simulink model "Motor_model"  (R2024b)
settings: Solver=FixedStepDiscrete  StartTime=0.0  StopTime=10  FixedStep=0.001  RelTol=1e-3
settings Model: Creator=divg2  LastModifiedBy=divg2
settings RTWCC: GPUComputeCapability=3.5

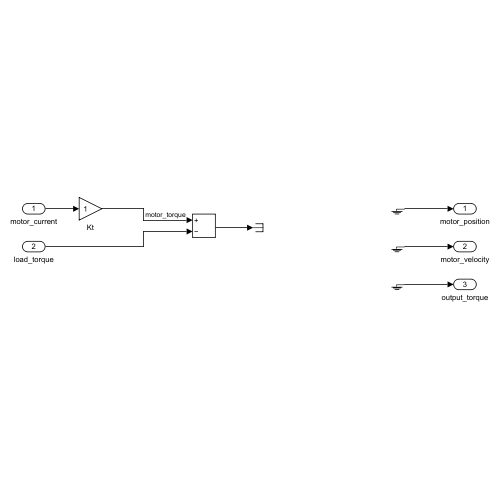
[thumbnail: Simulink's stored preview of the top-level diagram]
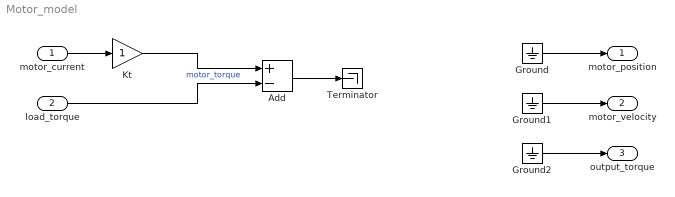
== system Motor_model ==
  motor_current : Inport
  load_torque : Inport  Port=2
  Add : Sum  Inputs=+-
  Ground : Ground
  Ground1 : Ground
  Ground2 : Ground
  Kt : Gain
  Terminator : Terminator
  motor_position : Outport
  motor_velocity : Outport  Port=2
  output_torque : Outport  Port=3
  wires:
  motor_current/1 -> Kt/1
  Ground/1 -> motor_position/1
  Ground1/1 -> motor_velocity/1
  Ground2/1 -> output_torque/1
  Kt/1 -> Add/1  "motor_torque"
  load_torque/1 -> Add/2
  Add/1 -> Terminator/1
